simulink model "Truck_ACC_Project"  (R2026a)
settings: Solver=ode4  StopTime=60  FixedStep=0.01
settings Model: Creator=adhav  LastModifiedBy=adhav

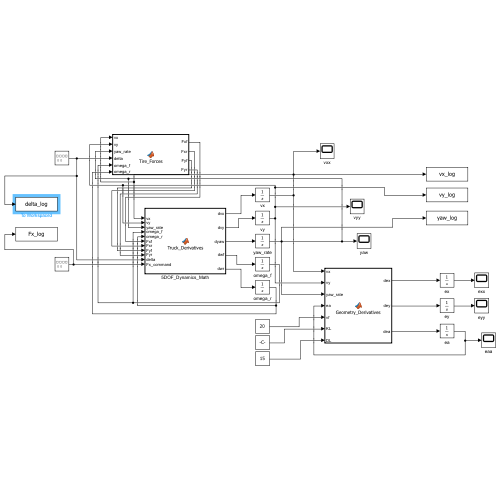
[thumbnail: Simulink's stored preview of the top-level diagram]
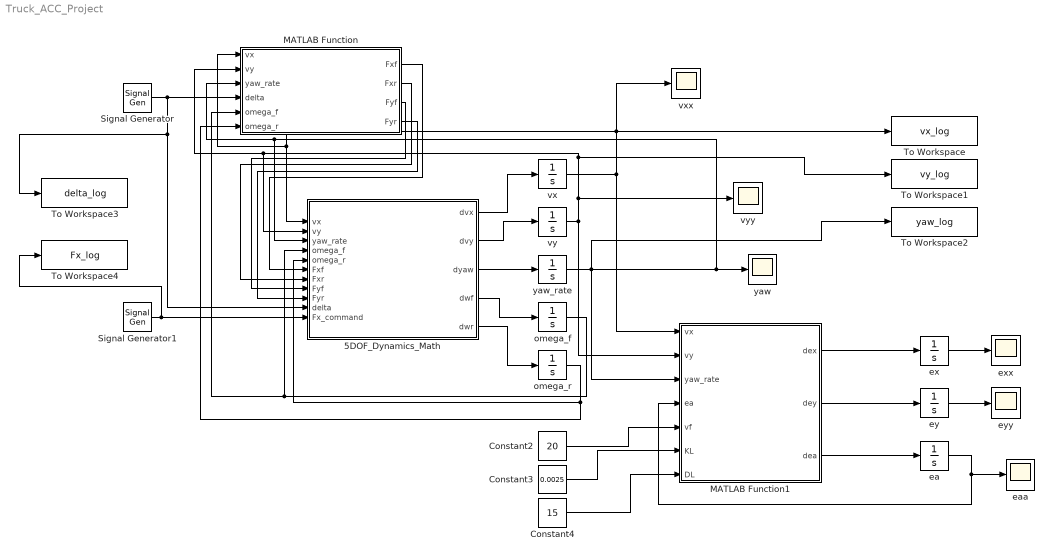
== system Truck_ACC_Project ==
  5DOF_Dynamics_Math : MATLAB Function  TreatAsAtomicUnit=on
  Constant2 : Constant  Value=20
  Constant3 : Constant  Value=0.0025
  Constant4 : Constant  Value=15
  MATLAB Function : MATLAB Function  TreatAsAtomicUnit=on
  MATLAB Function1 : MATLAB Function  TreatAsAtomicUnit=on
  Signal Generator : SignalGenerator  Amplitude=4  Frequency=0.2  Units=rad/sec
  Signal Generator1 : SignalGenerator  Amplitude=4000  Frequency=0.1  Units=rad/sec
  To Workspace : ToWorkspace  VariableName=vx_log  SampleTime=-1
  To Workspace1 : ToWorkspace  VariableName=vy_log  SampleTime=-1
  To Workspace2 : ToWorkspace  VariableName=yaw_log  SampleTime=-1
  To Workspace3 : ToWorkspace  VariableName=delta_log  SampleTime=-1
  To Workspace4 : ToWorkspace  VariableName=Fx_log  SampleTime=-1
  ea : Integrator
  eaa : Scope
      settings: ActiveDisplayYMinimum=-6.7292824196365606  ActiveDisplayYMaximum=5.4180734781565132  DataLoggingVariableName=ScopeData5
  ex : Integrator
  exx : Scope
      settings: ActiveDisplayYMinimum=-21.727446032725027  ActiveDisplayYMaximum=59.717552445964671  DataLoggingVariableName=ScopeData3
  ey : Integrator
  eyy : Scope
      settings: ActiveDisplayYMinimum=-1  ActiveDisplayYMaximum=1  DataLoggingVariableName=ScopeData4
  omega_f : Integrator  InitialCondition=16 / 0.51
  omega_r : Integrator  InitialCondition=31.37
  vx : Integrator  InitialCondition=16
  vxx : Scope
      settings: ActiveDisplayYMinimum=13.422691145228319  ActiveDisplayYMaximum=16.772175941768666
  vy : Integrator
  vyy : Scope
      settings: ActiveDisplayYMinimum=-1.5068497535434187  ActiveDisplayYMaximum=17.065554681695488  DataLoggingVariableName=ScopeData2
  yaw : Scope
      settings: ActiveDisplayYMinimum=-0.5801652367393253  ActiveDisplayYMaximum=0.1796896746259507
  yaw_rate : Integrator
  wires:
  5DOF_Dynamics_Math/1(dvx) -> vx/1
  5DOF_Dynamics_Math/2(dvy) -> vy/1
  5DOF_Dynamics_Math/4(dwf) -> omega_f/1
  5DOF_Dynamics_Math/3(dyaw) -> yaw_rate/1
  5DOF_Dynamics_Math/5(dwr) -> omega_r/1
  vx/1 -> MATLAB Function1/1(vx), vxx/1, To Workspace/1, MATLAB Function/1(vx), 5DOF_Dynamics_Math/1(vx)
  yaw_rate/1 -> To Workspace2/1, MATLAB Function1/3(yaw_rate), MATLAB Function/3(yaw_rate), 5DOF_Dynamics_Math/3(yaw_rate), yaw/1
  omega_f/1 -> MATLAB Function/5(omega_f), 5DOF_Dynamics_Math/4(omega_f)
  omega_r/1 -> MATLAB Function/6(omega_r), 5DOF_Dynamics_Math/5(omega_r)
  MATLAB Function/1(Fxf) -> 5DOF_Dynamics_Math/6(Fxf)
  MATLAB Function/2(Fxr) -> 5DOF_Dynamics_Math/7(Fxr)
  MATLAB Function/3(Fyf) -> 5DOF_Dynamics_Math/8(Fyf)
  MATLAB Function/4(Fyr) -> 5DOF_Dynamics_Math/9(Fyr)
  Signal Generator/1 -> MATLAB Function/4(delta), To Workspace3/1, 5DOF_Dynamics_Math/10(delta)
  Signal Generator1/1 -> To Workspace4/1, 5DOF_Dynamics_Math/11(Fx_command)
  MATLAB Function1/1(dex) -> ex/1
  MATLAB Function1/2(dey) -> ey/1
  MATLAB Function1/3(dea) -> ea/1
  ea/1 -> eaa/1, MATLAB Function1/4(ea)
  Constant2/1 -> MATLAB Function1/5(vf)
  Constant3/1 -> MATLAB Function1/6(KL)
  Constant4/1 -> MATLAB Function1/7(DL)
  ey/1 -> eyy/1
  ex/1 -> exx/1
  vy/1 -> vyy/1, MATLAB Function/2(vy), 5DOF_Dynamics_Math/2(vy), To Workspace1/1, MATLAB Function1/2(vy)

== matlab function Truck_ACC_Project/5DOF_Dynamics_Math ==
  data: vx input; dvx output; vy input; yaw_rate input; omega_f input; omega_r input; Fxf input; Fxr input; Fyf input; Fyr input; delta input; Fx_command input; dvy output; dyaw output; dwf output; dwr output
function [dvx, dvy, dyaw, dwf, dwr] = Truck_Derivatives(vx, vy, yaw_rate, omega_f, omega_r, Fxf, Fxr, Fyf, Fyr, delta, Fx_command)
% 5DOF TRUCK DYNAMICS (Equation 31)
% Calculates the derivatives (accelerations) of the truck states.

    %% Parameters (From Table IV)
    m = 18000;      % Mass (kg)
    a = 3.5;        % Front axle to CoM (m)
    b = 1.5;        % Rear axle to CoM (m)
    Iz = 130421;    % Yaw moment of inertia (kg*m^2)
    Jf = 24;        % Front wheel inertia (kg*m^2)
    Jr = 48;        % Rear wheel inertia (kg*m^2)
    Re = 0.51;      % Wheel rolling radius (m)
    
    %% Unit Conversions
    delta_rad = deg2rad(delta); % Steering angle to radians
    
    % The control input is a longitudinal Force (Fx). 
    % Equation 31 requires Drive Torques (Tdf, Tdr). 
    % We convert Force to Torque: Torque = Force * Radius. 
    % We split the total force 50/50 to front and rear wheels.
    Tdf = (Fx_command * Re) / 2;  
    Tdr = (Fx_command * Re) / 2;  

    %% Equation 31 (Ignoring aerodynamic drag for now as parameters aren't in the paper)
    % 1. Longitudinal velocity derivative (dvx)
    dvx = (vy * yaw_rate) + ((Fxf * cos(delta_rad) - Fyf * sin(delta_rad) + Fxr) / m);
    
    % 2. Lateral velocity derivative (dvy)
    dvy = (-vx * yaw_rate) + ((Fxf * sin(delta_rad) + Fyf * cos(delta_rad) + Fyr) / m);
    
    % 3. Yaw rate derivative (dyaw)
    dyaw = ((Fxf * sin(delta_rad) + Fyf * cos(delta_rad)) * a - Fyr * b) / Iz;
    
    % 4. Front wheel rotational derivative (dwf)
    dwf = (Tdf - Re * Fxf) / Jf;
    
    % 5. Rear wheel rotational derivative (dwr)
    dwr = (Tdr - Re * Fxr) / Jr;
end

== matlab function Truck_ACC_Project/MATLAB Function ==
  data: vx input; Fxf output; vy input; yaw_rate input; delta input; omega_f input; omega_r input; Fxr output; Fyf output; Fyr output
function [Fxf, Fxr, Fyf, Fyr] = Tire_Forces(vx, vy, yaw_rate, delta, omega_f, omega_r)
% MAGIC FORMULA TIRE MODEL
% Translates Equations 32 and 33 from the IEEE paper using Tables III & IV.

    %% 1. Define Parameters (From Table IV)
    a = 3.5;      % Front wheel to center of mass distance (m)
    b = 1.5;      % Rear wheel to center of mass distance (m)
    Re = 0.51;    % Wheel rolling radius (m)
    
    %% 2. Define Tire Parameters (From Table III)
    % Longitudinal Forces (Fxf, Fxr)
    B_kf = 8.61;  C_kf = 1.58;  D_kf = 22053;  E_kf = 0.5624;
    B_kr = 8.61;  C_kr = 1.58;  D_kr = 44625;  E_kr = 0.5624;
    
    % Lateral Forces (Fyf, Fyr)
    B_af = 6.59;  C_af = 2.42;  D_af = 22053;  E_af = -0.3028;
    B_ar = 6.59;  C_ar = 2.42;  D_ar = 44625;  E_ar = -0.3028;
    
    %% 3. Unit Conversions
    % delta is constrained to [-10, 10] degrees in the paper, convert to radians
    delta_rad = deg2rad(delta); 
    
    % Safety buffer to prevent division by zero
    epsilon = 1e-6; 

    %% 4. Calculate Slip Ratios (Equation 32)
    kf = (omega_f * Re - vx) / max(omega_f * Re, vx + epsilon);
    kr = (omega_r * Re - vx) / max(omega_r * Re, vx + epsilon);

    %% 5. Calculate Slip Angles (Equation 33)
    % Determine tire longitudinal and lateral velocities
    v_alpha_f = vx * cos(delta_rad) + (vy + a * yaw_rate) * sin(delta_rad);
    v_beta_f  = (vy + a * yaw_rate) * cos(delta_rad) - vx * sin(delta_rad);
    
    v_alpha_r = vx;
    v_beta_r  = vy - b * yaw_rate;
    
    % Calculate slip angles
    alpha_f = sign(v_alpha_f) * atan(v_beta_f / (abs(v_alpha_f) + epsilon));
    alpha_r = sign(v_alpha_r) * atan(v_beta_r / (abs(v_alpha_r) + epsilon));

    %% 6. Magic Formula Equation (Bottom of Section IV-A)
    % Front Longitudinal Force (Fxf)
    Fxf = D_kf * sin(C_kf * atan(B_kf * kf - E_kf * (B_kf * kf - atan(B_kf * kf))));
    
    % Rear Longitudinal Force (Fxr)
    Fxr = D_kr * sin(C_kr * atan(B_kr * kr - E_kr * (B_kr * kr - atan(B_kr * kr))));
    
    % Front Lateral Force (Fyf)
    Fyf = D_af * sin(C_af * atan(B_af * alpha_f - E_af * (B_af * alpha_f - atan(B_af * alpha_f))));
    
    % Rear Lateral Force (Fyr)
    Fyr = D_ar * sin(C_ar * atan(B_ar * alpha_r - E_ar * (B_ar * alpha_r - atan(B_ar * alpha_r))));
end

== matlab function Truck_ACC_Project/MATLAB Function1 ==
  data: vx input; dex output; vy input; yaw_rate input; ea input; vf input; KL input; DL input; dey output; dea output
function [dex, dey, dea] = Geometry_Derivatives(vx, vy, yaw_rate, ea, vf, KL, DL)
% LANE-KEEPING & ACC GEOMETRY (Equations 18, 19, 20)
% Calculates the rate of change of errors.

    %% Equation 20: Longitudinal position error derivative
    % e_dot_x = v_f - v_x
    dex = vf - vx;
    
    %% Equation 18b: Heading angle error derivative
    % e_dot_a = v_x * K_L - yaw_rate
    dea = vx * KL - yaw_rate;
    
    %% Equation 18a: Lateral position error derivative
    % e_dot_y = v_x * e_a - v_y - yaw_rate * D_L
    dey = vx * ea - vy - yaw_rate * DL;
end
